simulink model "IPMSM_Motor_Drive1"  (R2022b)
settings: Solver=VariableStepAuto  StartTime=0.0  StopTime=10.0  RelTol=1e-3
InitFcn:
  | Ts=1/(16000);
  | Ts_Control=Ts;
  | Ts_Power=Ts;
  | PulseDuration=5e-6;
  | Vrefpeak=399;
  | VDC=800;
  | R=1.4;
  | L=1e-4;
  | Freq = 120;
  | Rc= 0.00001;
  | C=220e-6;
  | Ld = 473e-6;
  | Lq = 1155e-6;
  | Fpm = 0.1383;
  | Rs = 0.036;
libraries: spsIGBTDiodeLib x12, spsDiodeLib x6, spsSeriesRLCBranchLib x3, slpidlib x2, spsDCVoltageSourceLib x1, mcbcontrolslib x1, spsPermanentMagnetSynchronousMachineLib x1, simulink x1, spsThreePhaseVIMeasurementLib x1, spspowerguiLib x1
settings Model: Creator=ahmetcan.akuz  LastModifiedBy=ahmetcan.akuz

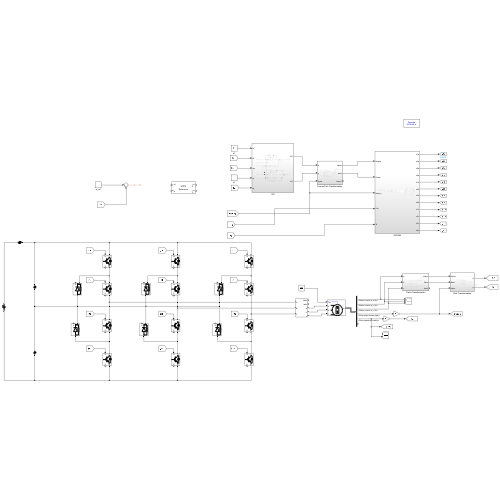
[thumbnail: Simulink's stored preview of the top-level diagram]
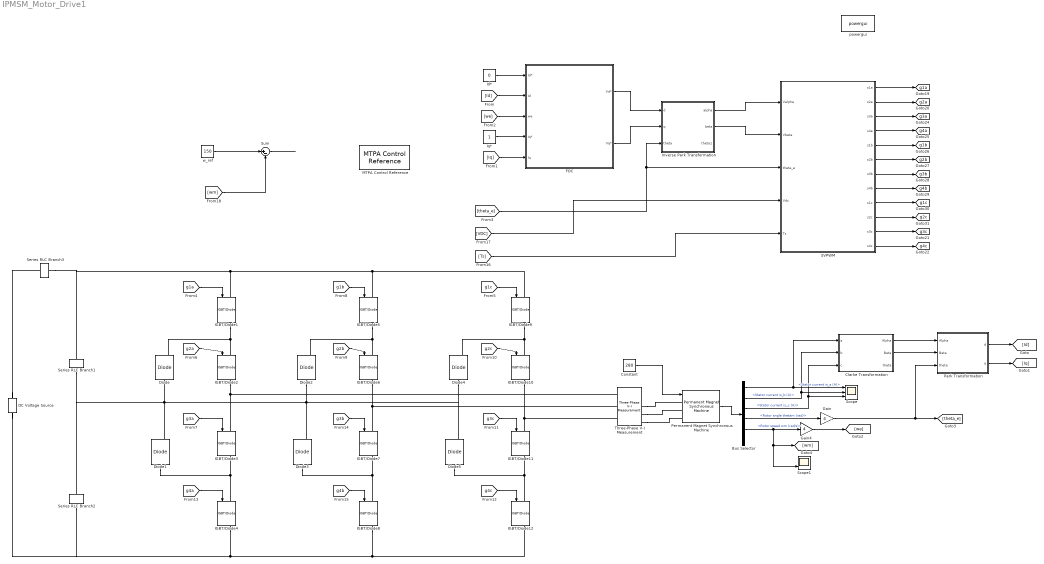
== system IPMSM_Motor_Drive1 ==
  Bus Selector : BusSelector  OutputSignals=Stator current is_a (A),Stator current is_b (A),Stator current is_c (A),Rotor angle thetam (rad),Rotor speed wm (rad/s),Electromagnetic torque Te (N*m)
  Clarke Transformation : Subsystem
  Constant : Constant  Value=280
  DC Voltage Source : spsDCVoltageSourceLib/DC Voltage Source  Amplitude=800  Measurements=None
  Diode{,1..5} (6 alike) : spsDiodeLib/Diode  Ron=1e-5  Lon=0  Vf=0.8  IC=0  UseSnubber=0  Rs=1e6  Cs=inf  Measurements=on
  FOC : Subsystem
  Gain : Gain  Gain=4
  Gain4 : Gain  Gain=4
  IGBT/Diode{1..12} (12 alike) : spsIGBTDiodeLib/IGBT//Diode  Ron=1e-3  Rs=1e5  Cs=inf  Measurements=on
  Id* : Constant  Value=0
  Inverse Park Transformation : Subsystem
  Iq* : Constant
  MTPA Control Reference : mcbcontrolslib/MTPA Control Reference  VariantSelect=Interior PMSM  polePairs=4  Rs=0.36  Ld=0.2e-3  Lq=0.4e-3  FluxPM=6.4e-3  ilimit=7.1  V_dc=24  Units=Per-Unit (PU)  N_base=4107  I_base=19.3  T_base=0.74112  N_base_disp=3182
      settings: LibrarySourceBlock=mcblib/Controls/Control Reference/MTPA Control Reference
  Park Transformation : Subsystem
  Permanent Magnet Synchronous Machine : spsPermanentMagnetSynchronousMachineLib/Permanent Magnet Synchronous Machine  NbPhases=3  FluxDistribution=Sinusoidal  RotorType=Salient-pole  MechanicalLoad=Torque Tm  PresetModel=No  ShowDetailedParameters=on  MeasurementBus=off  Resistance=0.036  Inductance=8.5e-3  dqInductances=[0.473e-3,1.155e-3]  La=0.000395  MachineConstant=Flux linkage established by magnets (V.s)  Flux=0.1383  VoltageCst=100.3394  TorqueCst=0.8298  Flat=120  Mechanical=[0.0027 0.0004924 4 0]  PolePairs=4  InitialConditions=[0,0, 0,0]  InitialConditions5ph=[0 0 0 0 0 0]  RefAngle=Aligned with phase A axis (original Park)  IterativeDiscreteModel=Trapezoidal non iterative  TsBlock=-1  TsPowergui=0
  SVPWM : Subsystem
  Scope : Scope  NumInputPorts=3
  Scope1 : Scope  NumInputPorts=2
  Series RLC Branch1 : spsSeriesRLCBranchLib/Series RLC Branch  LConnTagsString=__new0  RConnTagsString=__new0  BranchType=C  Resistance=1e-3  Inductance=1e-3  SetiL0=off  InitialCurrent=0  Capacitance=500e-6  Setx0=on  InitialVoltage=800/2  Measurements=Branch voltage
  Series RLC Branch2 : spsSeriesRLCBranchLib/Series RLC Branch  LConnTagsString=__new0  RConnTagsString=__new0  BranchType=C  Resistance=1e-3  Inductance=1e-3  SetiL0=off  InitialCurrent=0  Capacitance=500e-6  Setx0=on  InitialVoltage=800/2  Measurements=Branch voltage
  Series RLC Branch3 : spsSeriesRLCBranchLib/Series RLC Branch  LConnTagsString=__new0  RConnTagsString=__new0  BranchType=R  Resistance=1e-3  Inductance=1e-3  SetiL0=off  InitialCurrent=0  Capacitance=500e-6  Setx0=on  InitialVoltage=800/2  Measurements=Branch voltage
  Sum : Sum  Inputs=|+-
  Three-Phase V-I Measurement : spsThreePhaseVIMeasurementLib/Three-Phase V-I Measurement  VoltageMeasurement=phase-to-phase  SetLabelV=off  LabelV=Vabc  Vpu=off  VpuLL=off  CurrentMeasurement=yes  SetLabelI=off  LabelI=Iabc  Ipu=off  Pbase=100e6  Vbase=500e3  OutputType=Complex  PhasorSimulation=off  PSBequivalent=0
  powergui : spspowerguiLib/powergui  Priority=1  SimulationMode=Discrete  SampleTime=Ts/10  frequency=60  Iterations=50  frequencyindice=0  Pbase=100e6  ErrMax=1e-4  UnitsV=kV  UnitsW=MW  buscounter=0  FunctionMessages=off  echomessages=off  EnableUseOfTLC=off  CurrentSourceSwitches=off  DisableSnubberDevices=off  DisableRonSwitches=off  DisableVfSwitches=off  DisplayEquations=off  AutomaticDiscreteSolvers=off  SolverType=Tustin/Backward Euler (TBE)  Interpol=off  ExternalGateDelay=off  methode=off  Ts=100  x0status=blocks  SPID=off  SwTol=0  HookPort=off  NonlinearTolerance=1e-4  nMaxIteration=100  ContinueOnMaxIteration=off  RestoreLinks=warning  ResistiveCurrentMeasurement=off  Frange=[0:2:500]  Ylog=off  Xlog=on  ShowGrid=off  save=off  variable=ZData  structure=0  ZoomFFT=off  StartTime=0.0  cycles=1  DisplayStyle=1  fundamental=60  FreqAxis=off  MaxFrequency=1000  frequencyindicesteady=1  RmsSteady=1  display=off
  w_ref : Constant  Value=150
  tag scope: g1a=global, g1b=global, g1c=global, g2a=global, g2b=global, g2c=global, g3a=global, g3b=global, g3c=global, g4a=global, g4b=global, g4c=global
  wires:
  Permanent Magnet Synchronous Machine/1 -> Bus Selector/1
  Bus Selector/1 -> Scope/1, Clarke Transformation/1(a)  "<Stator current is_a (A)>"
  Bus Selector/2 -> Clarke Transformation/2(b), Scope/2  "<Stator current is_b (A)>"
  Bus Selector/3 -> Clarke Transformation/3(c), Scope/3  "<Stator current is_c (A)>"
  Clarke Transformation/2(Beta) -> Park Transformation/2(Beta)
  Clarke Transformation/1(Alpha) -> Park Transformation/1(Alpha)
  Bus Selector/4 -> Gain/1  "<Rotor angle thetam (rad)>"
  Gain/1 -> [theta_e], Park Transformation/3(theta)
  Park Transformation/1(d) -> [Id]
  Park Transformation/2(q) -> [Iq]
  Bus Selector/5 -> [wm], Scope1/2, Gain4/1  "<Rotor speed wm (rad/s)>"
  Gain4/1 -> [we]
  Id*/1 -> FOC/1(Id*)
  [Id] -> FOC/2(Id)
  [we] -> FOC/3(we)
  Iq*/1 -> FOC/4(Iq*)
  [Iq] -> FOC/5(Iq)
  FOC/1(Vd*) -> Inverse Park Transformation/1(d)
  FOC/2(Vq*) -> Inverse Park Transformation/2(q)
  [theta_e] -> SVPWM/3(theta_e), Inverse Park Transformation/3(theta)
  Inverse Park Transformation/1(alpha) -> SVPWM/1(Valpha)
  Inverse Park Transformation/2(beta) -> SVPWM/2(Vbeta)
  [g1a] -> IGBT/Diode1/1
  [g2b] -> IGBT/Diode6/1
  [g3b] -> IGBT/Diode7/1
  [g4b] -> IGBT/Diode8/1
  [g4a] -> IGBT/Diode4/1
  [g3a] -> IGBT/Diode3/1
  [g2a] -> IGBT/Diode2/1
  [g1b] -> IGBT/Diode5/1
  [g1c] -> IGBT/Diode9/1
  [g2c] -> IGBT/Diode10/1
  [g3c] -> IGBT/Diode11/1
  [g4c] -> IGBT/Diode12/1
  SVPWM/1(s1a) -> [g1a]
  SVPWM/2(s2a) -> [g2a]
  SVPWM/12(s4c) -> [g4c]
  SVPWM/11(s3c) -> [g3c]
  SVPWM/3(s3a) -> [g3a]
  SVPWM/4(s4a) -> [g4a]
  SVPWM/5(s1b) -> [g1b]
  SVPWM/6(s2b) -> [g2b]
  SVPWM/7(s3b) -> [g3b]
  SVPWM/8(s4b) -> [g4b]
  SVPWM/9(s1c) -> [g1c]
  SVPWM/10(s2c) -> [g2c]
  [Ts] -> SVPWM/5(Ts)
  [VDC] -> SVPWM/4(Vdc)
  Constant/1 -> Permanent Magnet Synchronous Machine/1
  w_ref/1 -> Sum/1
  [wm] -> Sum/2
  Sum/1 -> ?
  connections:
  Diode1/RConn1 -- Series RLC Branch1/RConn1 -- Series RLC Branch2/LConn1 -- Diode3/RConn1 -- Diode5/RConn1 -- Diode4/LConn1 -- Diode2/LConn1 -- Diode/LConn1
  IGBT/Diode4/LConn1 -- Diode1/LConn1 -- IGBT/Diode3/RConn1
  IGBT/Diode2/RConn1 -- IGBT/Diode3/LConn1 -- Three-Phase V-I Measurement/LConn1
  IGBT/Diode1/RConn1 -- Diode/RConn1 -- IGBT/Diode2/LConn1
  IGBT/Diode5/RConn1 -- Diode2/RConn1 -- IGBT/Diode6/LConn1
  IGBT/Diode8/LConn1 -- Diode3/LConn1 -- IGBT/Diode7/RConn1
  IGBT/Diode6/RConn1 -- Three-Phase V-I Measurement/LConn2 -- IGBT/Diode7/LConn1
  IGBT/Diode9/RConn1 -- Diode4/RConn1 -- IGBT/Diode10/LConn1
  IGBT/Diode12/LConn1 -- Diode5/LConn1 -- IGBT/Diode11/RConn1
  IGBT/Diode10/RConn1 -- Three-Phase V-I Measurement/LConn3 -- IGBT/Diode11/LConn1
  IGBT/Diode1/LConn1 -- Series RLC Branch3/LConn1 -- Series RLC Branch1/LConn1 -- IGBT/Diode9/LConn1 -- IGBT/Diode5/LConn1
  IGBT/Diode4/RConn1 -- Series RLC Branch2/RConn1 -- DC Voltage Source/LConn1 -- IGBT/Diode8/RConn1 -- IGBT/Diode12/RConn1
  Three-Phase V-I Measurement/RConn3 -- Permanent Magnet Synchronous Machine/LConn3
  Three-Phase V-I Measurement/RConn2 -- Permanent Magnet Synchronous Machine/LConn2
  Three-Phase V-I Measurement/RConn1 -- Permanent Magnet Synchronous Machine/LConn1
  DC Voltage Source/RConn1 -- Series RLC Branch3/RConn1

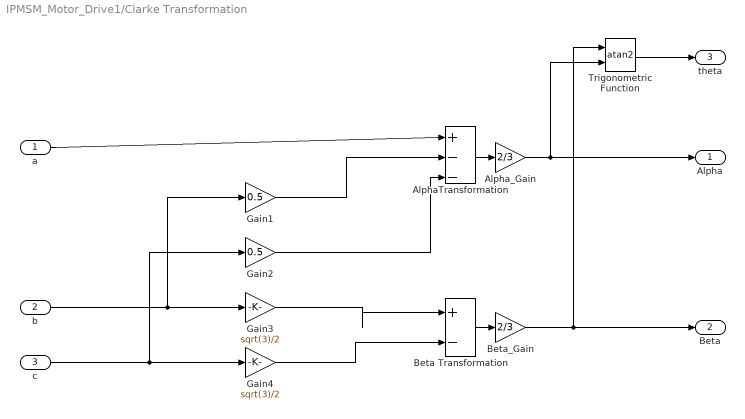
== system IPMSM_Motor_Drive1/Clarke Transformation ==
  a : Inport
  b : Inport  Port=2
  c : Inport  Port=3
  AlphaTransformation : Sum  Inputs=|+--
  Alpha_Gain : Gain  Gain=2/3
  Beta Transformation : Sum  Inputs=|+-
  Beta_Gain : Gain  Gain=2/3
  Gain1 : Gain  Gain=0.5
  Gain2 : Gain  Gain=0.5
  Gain3 : Gain  Gain=sqrt(3)/2
  Gain4 : Gain  Gain=sqrt(3)/2
  Trigonometric Function : Trigonometry  Operator=atan2
  Alpha : Outport
  Beta : Outport  Port=2
  theta : Outport  Port=3
  wires:
  Gain1/1 -> AlphaTransformation/2
  Gain4/1 -> Beta Transformation/2
  AlphaTransformation/1 -> Alpha_Gain/1
  Gain3/1 -> Beta Transformation/1
  b/1 -> Gain1/1, Gain3/1
  Gain2/1 -> AlphaTransformation/3
  c/1 -> Gain2/1, Gain4/1
  Beta Transformation/1 -> Beta_Gain/1
  a/1 -> AlphaTransformation/1
  Trigonometric Function/1 -> theta/1
  Alpha_Gain/1 -> Trigonometric Function/2, Alpha/1
  Beta_Gain/1 -> Trigonometric Function/1, Beta/1

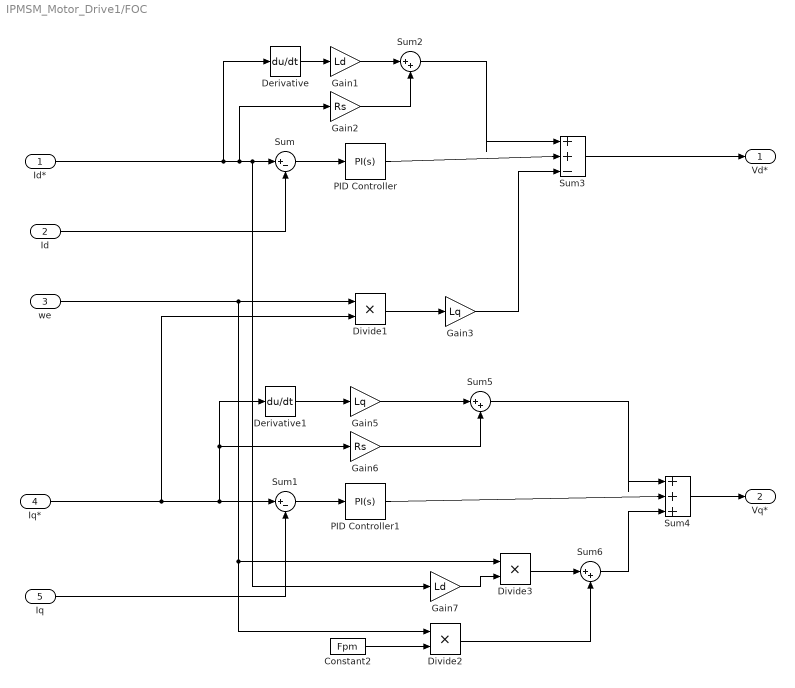
== system IPMSM_Motor_Drive1/FOC ==
  Id* : Inport
  Id : Inport  Port=2
  we : Inport  Port=3
  Iq* : Inport  Port=4
  Iq : Inport  Port=5
  Constant2 : Constant  Value=Fpm
  Derivative : Derivative
  Derivative1 : Derivative
  Divide1 : Product  Inputs=**
  Divide2 : Product  Inputs=**
  Divide3 : Product  Inputs=**
  Gain1 : Gain  Gain=Ld
  Gain2 : Gain  Gain=Rs
  Gain3 : Gain  Gain=Lq
  Gain5 : Gain  Gain=Lq
  Gain6 : Gain  Gain=Rs
  Gain7 : Gain  Gain=Ld
  PID Controller : slpidlib/PID Controller  Controller=PI  Form=Parallel  TimeDomain=Continuous-time  UseExternalTs=off  SampleTime=-1  IntegratorMethod=Forward Euler  FilterMethod=Forward Euler  ControllerParametersSource=internal  P=1  I=1  UseKiTs=off  D=0  N=100  UseFilter=on  TunerSelectOption=Transfer Function Based (PID Tuner App)  InitialConditionSource=internal  InitialConditionForIntegrator=0  InitialConditionForFilter=0  DifferentiatorICPrevScaledInput=0  ExternalReset=none  TrackingMode=off  Kt=1  LimitOutput=off  SatLimitsSource=internal  UpperSaturationLimit=inf  LowerSaturationLimit=-inf  LinearizeAsGain=on  AntiWindupMode=none  Kb=1  LimitIntegrator=off  UpperIntegratorSaturationLimit=inf  LowerIntegratorSaturationLimit=-inf  POutMin=[]  POutMax=[]  IOutMin=[]  IOutMax=[]  DOutMin=[]  DOutMax=[]  NOutMin=[]  NOutMax=[]  SumOutMin=[]  SumOutMax=[]  SaturationOutMin=[]  SaturationOutMax=[]  PParamMin=[]  PParamMax=[]  IParamMin=[]  IParamMax=[]  DParamMin=[]  DParamMax=[]  NParamMin=[]  NParamMax=[]  KbParamMin=[]  KbParamMax=[]  KtParamMin=[]  KtParamMax=[]  KbOutMin=[]  KbOutMax=[]  KtOutMin=[]  KtOutMax=[]  IntegratorOutMin=[]  IntegratorOutMax=[]  FilterOutMin=[]  FilterOutMax=[]  SumI1OutMin=[]  SumI1OutMax=[]  SumI2OutMin=[]  SumI2OutMax=[]  SumI3OutMin=[]  SumI3OutMax=[]  SumI4OutMin=[]  SumI4OutMax=[]  SumDOutMin=[]  SumDOutMax=[]  DifferentiatorOutMin=[]  DifferentiatorOutMax=[]  FilterDiffOutCoefMin=[]  FilterDiffOutCoefMax=[]  ReciprocalOutMin=[]  ReciprocalOutMax=[]  SumDenOutMin=[]  SumDenOutMax=[]  SumNumOutMin=[]  SumNumOutMax=[]  DivideOutMin=[]  DivideOutMax=[]  UdiffTsProdOutMin=[]  UdiffTsProdOutMax=[]  NTsProdOutMin=[]  NTsProdOutMax=[]  UintegralTsProdOutMin=[]  UintegralTsProdOutMax=[]  UngainTsProdOutMin=[]  UngainTsProdOutMax=[]  ClampingZeroOutDataTypeStr=Inherit: Inherit via back propagation  ClampingZeroOutMin=[]  ClampingZeroOutMax=[]  FilterDenConstantOutDataTypeStr=Inherit: Inherit via back propagation  FilterDenConstantOutMin=[]  FilterDenConstantOutMax=[]  PCopyOutDataTypeStr=Inherit: Inherit via back propagation  PCopyOutMin=[]  PCopyOutMax=[]  NCopyOutDataTypeStr=Inherit: Inherit via back propagation  NCopyOutMin=[]  NCopyOutMax=[]  IntegratorContinuousStateAttributes=''  IntegratorStateMustResolveToSignalObject=off  IntegratorRTWStateStorageClass=Auto  FilterContinuousStateAttributes=''  FilterStateMustResolveToSignalObject=off  FilterRTWStateStorageClass=Auto  ParallelPVariant=InternalParameters  IdealPVariant=Disabled  IVariant=InternalParameters  DVariant=Disabled  IntegratorVariant=Continuous  SatVariant=Disabled  AWVariant=Passthrough  PCopyVariant=Disabled  TRVariant=Disabled  FdbkBlocksVariant=Forward  IdealPFdbkVariant=Disabled  SatFdbkVariant=Disabled  DerivativeFilterVariant=Disabled  NVariant=Disabled  NCopyVariant=Disabled_SignalSpec  FilterICVariant=Disabled  IntegratorICVariant=InternalICs  ExternalResetVariant=Disabled  TRSumVariant=Passthrough  SumFdbkVariant=Disabled  SumVariant=Sum_PI  TsampFilterVariant=InternalTs  TsampNgainVariant=Passthrough  TsampIntegralVariant=Passthrough  ExternalSaturationOutDataTypeStr=Inherit: Same as second input
  PID Controller1 : slpidlib/PID Controller  Controller=PI  Form=Parallel  TimeDomain=Continuous-time  UseExternalTs=off  SampleTime=-1  IntegratorMethod=Forward Euler  FilterMethod=Forward Euler  ControllerParametersSource=internal  P=1  I=1  UseKiTs=off  D=0  N=100  UseFilter=on  TunerSelectOption=Transfer Function Based (PID Tuner App)  InitialConditionSource=internal  InitialConditionForIntegrator=0  InitialConditionForFilter=0  DifferentiatorICPrevScaledInput=0  ExternalReset=none  TrackingMode=off  Kt=1  LimitOutput=off  SatLimitsSource=internal  UpperSaturationLimit=inf  LowerSaturationLimit=-inf  LinearizeAsGain=on  AntiWindupMode=none  Kb=1  LimitIntegrator=off  UpperIntegratorSaturationLimit=inf  LowerIntegratorSaturationLimit=-inf  POutMin=[]  POutMax=[]  IOutMin=[]  IOutMax=[]  DOutMin=[]  DOutMax=[]  NOutMin=[]  NOutMax=[]  SumOutMin=[]  SumOutMax=[]  SaturationOutMin=[]  SaturationOutMax=[]  PParamMin=[]  PParamMax=[]  IParamMin=[]  IParamMax=[]  DParamMin=[]  DParamMax=[]  NParamMin=[]  NParamMax=[]  KbParamMin=[]  KbParamMax=[]  KtParamMin=[]  KtParamMax=[]  KbOutMin=[]  KbOutMax=[]  KtOutMin=[]  KtOutMax=[]  IntegratorOutMin=[]  IntegratorOutMax=[]  FilterOutMin=[]  FilterOutMax=[]  SumI1OutMin=[]  SumI1OutMax=[]  SumI2OutMin=[]  SumI2OutMax=[]  SumI3OutMin=[]  SumI3OutMax=[]  SumI4OutMin=[]  SumI4OutMax=[]  SumDOutMin=[]  SumDOutMax=[]  DifferentiatorOutMin=[]  DifferentiatorOutMax=[]  FilterDiffOutCoefMin=[]  FilterDiffOutCoefMax=[]  ReciprocalOutMin=[]  ReciprocalOutMax=[]  SumDenOutMin=[]  SumDenOutMax=[]  SumNumOutMin=[]  SumNumOutMax=[]  DivideOutMin=[]  DivideOutMax=[]  UdiffTsProdOutMin=[]  UdiffTsProdOutMax=[]  NTsProdOutMin=[]  NTsProdOutMax=[]  UintegralTsProdOutMin=[]  UintegralTsProdOutMax=[]  UngainTsProdOutMin=[]  UngainTsProdOutMax=[]  ClampingZeroOutDataTypeStr=Inherit: Inherit via back propagation  ClampingZeroOutMin=[]  ClampingZeroOutMax=[]  FilterDenConstantOutDataTypeStr=Inherit: Inherit via back propagation  FilterDenConstantOutMin=[]  FilterDenConstantOutMax=[]  PCopyOutDataTypeStr=Inherit: Inherit via back propagation  PCopyOutMin=[]  PCopyOutMax=[]  NCopyOutDataTypeStr=Inherit: Inherit via back propagation  NCopyOutMin=[]  NCopyOutMax=[]  IntegratorContinuousStateAttributes=''  IntegratorStateMustResolveToSignalObject=off  IntegratorRTWStateStorageClass=Auto  FilterContinuousStateAttributes=''  FilterStateMustResolveToSignalObject=off  FilterRTWStateStorageClass=Auto  ParallelPVariant=InternalParameters  IdealPVariant=Disabled  IVariant=InternalParameters  DVariant=Disabled  IntegratorVariant=Continuous  SatVariant=Disabled  AWVariant=Passthrough  PCopyVariant=Disabled  TRVariant=Disabled  FdbkBlocksVariant=Forward  IdealPFdbkVariant=Disabled  SatFdbkVariant=Disabled  DerivativeFilterVariant=Disabled  NVariant=Disabled  NCopyVariant=Disabled_SignalSpec  FilterICVariant=Disabled  IntegratorICVariant=InternalICs  ExternalResetVariant=Disabled  TRSumVariant=Passthrough  SumFdbkVariant=Disabled  SumVariant=Sum_PI  TsampFilterVariant=InternalTs  TsampNgainVariant=Passthrough  TsampIntegralVariant=Passthrough  ExternalSaturationOutDataTypeStr=Inherit: Same as second input
  Sum : Sum  Inputs=|+-
  Sum1 : Sum  Inputs=|+-
  Sum2 : Sum  Inputs=|++
  Sum3 : Sum  Inputs=|++-
  Sum4 : Sum  Inputs=|+++
  Sum5 : Sum  Inputs=|++
  Sum6 : Sum  Inputs=|++
  Vd* : Outport
  Vq* : Outport  Port=2
  wires:
  Sum/1 -> PID Controller/1
  Iq*/1 -> Divide1/2, Gain6/1, Derivative1/1, Sum1/1
  Divide3/1 -> Sum6/1
  Id*/1 -> Derivative/1, Gain2/1, Gain7/1, Sum/1
  Derivative1/1 -> Gain5/1
  Sum6/1 -> Sum4/3
  Sum3/1 -> Vd*/1
  Gain7/1 -> Divide3/2
  Derivative/1 -> Gain1/1
  Gain1/1 -> Sum2/1
  PID Controller1/1 -> Sum4/2
  Gain2/1 -> Sum2/2
  Id/1 -> Sum/2
  Sum1/1 -> PID Controller1/1
  Sum5/1 -> Sum4/1
  Sum4/1 -> Vq*/1
  Gain6/1 -> Sum5/2
  PID Controller/1 -> Sum3/2
  Sum2/1 -> Sum3/1
  we/1 -> Divide3/1, Divide2/1, Divide1/1
  Iq/1 -> Sum1/2
  Divide2/1 -> Sum6/2
  Gain5/1 -> Sum5/1
  Constant2/1 -> Divide2/2
  Divide1/1 -> Gain3/1
  Gain3/1 -> Sum3/3

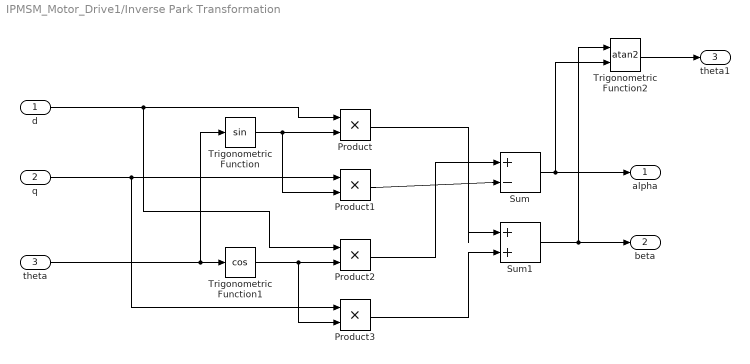
== system IPMSM_Motor_Drive1/Inverse Park Transformation ==
  d : Inport
  q : Inport  Port=2
  theta : Inport  Port=3
  Product{,1..3} (4 alike) : Product
  Sum : Sum  Inputs=|+-
  Sum1 : Sum  Inputs=|++
  Trigonometric Function : Trigonometry
  Trigonometric Function1 : Trigonometry  Operator=cos
  Trigonometric Function2 : Trigonometry  Operator=atan2
  alpha : Outport
  beta : Outport  Port=2
  theta1 : Outport  Port=3
  wires:
  Product/1 -> Sum1/1
  Trigonometric Function/1 -> Product1/2, Product/2
  d/1 -> Product2/1, Product/1
  Product2/1 -> Sum/1
  theta/1 -> Trigonometric Function/1, Trigonometric Function1/1
  Product1/1 -> Sum/2
  Trigonometric Function1/1 -> Product2/2, Product3/2
  q/1 -> Product3/1, Product1/1
  Product3/1 -> Sum1/2
  Sum/1 -> Trigonometric Function2/2, alpha/1
  Trigonometric Function2/1 -> theta1/1
  Sum1/1 -> Trigonometric Function2/1, beta/1

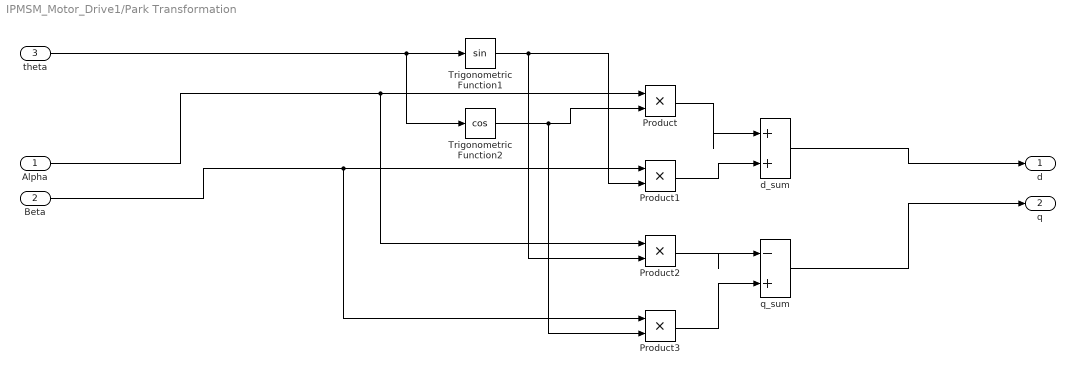
== system IPMSM_Motor_Drive1/Park Transformation ==
  Alpha : Inport
  Beta : Inport  Port=2
  theta : Inport  Port=3
  Product{,1..3} (4 alike) : Product
  Trigonometric Function1 : Trigonometry
  Trigonometric Function2 : Trigonometry  Operator=cos
  d_sum : Sum  Inputs=|++
  q_sum : Sum  Inputs=|-+
  d : Outport
  q : Outport  Port=2
  wires:
  Trigonometric Function1/1 -> Product2/2, Product1/2
  Product/1 -> d_sum/1
  Product2/1 -> q_sum/1
  Beta/1 -> Product3/1, Product1/1
  Alpha/1 -> Product2/1, Product/1
  Product3/1 -> q_sum/2
  Trigonometric Function2/1 -> Product3/2, Product/2
  Product1/1 -> d_sum/2
  q_sum/1 -> q/1
  d_sum/1 -> d/1
  theta/1 -> Trigonometric Function2/1, Trigonometric Function1/1

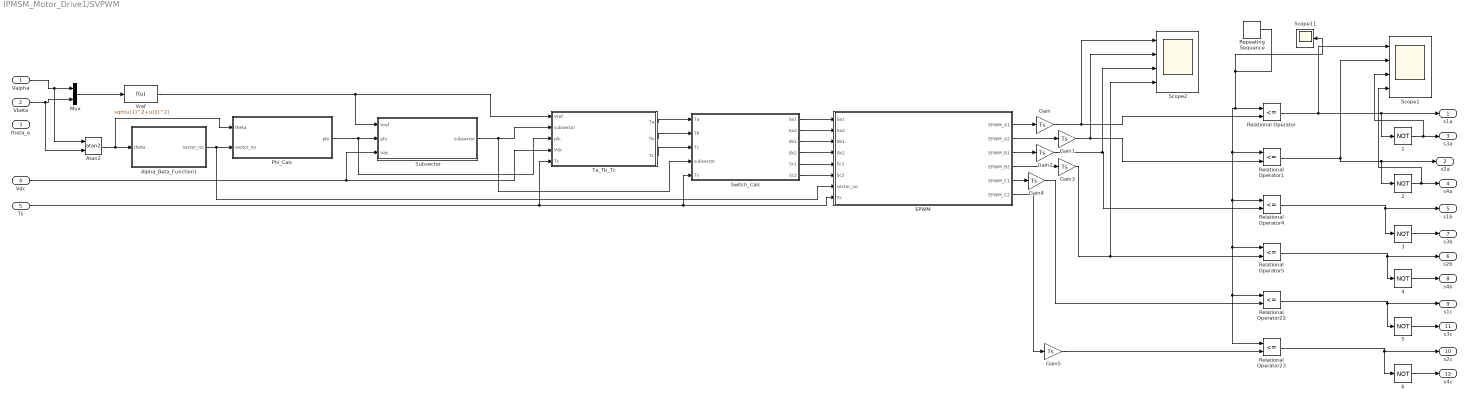
== system IPMSM_Motor_Drive1/SVPWM ==
  Valpha : Inport
  Vbeta : Inport  Port=2
  theta_e : Inport  Port=3
  Vdc : Inport  Port=4
  Ts : Inport  Port=5
  {1..6} (6 alike) : Logic  Operator=NOT  AllPortsSameDT=off  OutDataTypeStr=boolean
  Alpha_Beta_Function1 : MATLAB Function  TreatAsAtomicUnit=on
  Atan2 : Trigonometry  Operator=atan2
  EPWM : MATLAB Function  TreatAsAtomicUnit=on
  Gain{,1..5} (6 alike) : Gain  Gain=Ts
  Mux : Mux  Inputs=2
  Phi_Calc : MATLAB Function  TreatAsAtomicUnit=on
  Relational Operator{,1,4..5,22..23} (6 alike) : RelationalOperator  Operator=<=  OutDataTypeStr=boolean  InputSameDT=off
  Repeating Sequence : simulink/Sources/Repeating Sequence  rep_seq_t=[0 1 2]*[1/6000]  rep_seq_y=[0 0.01 0]
  Scope1 : Scope  NumInputPorts=4
  Scope11 : Scope
  Scope2 : Scope  NumInputPorts=4
  Subsector : MATLAB Function  TreatAsAtomicUnit=on
  Switch_Calc : MATLAB Function  TreatAsAtomicUnit=on
  Ta_Tb_Tc : MATLAB Function  TreatAsAtomicUnit=on
  Vref : Fcn  Expr=sqrt(u(1)^2+u(2)^2)
  s1a : Outport
  s2a : Outport  Port=2
  s3a : Outport  Port=3
  s4a : Outport  Port=4
  s1b : Outport  Port=5
  s2b : Outport  Port=6
  s3b : Outport  Port=7
  s4b : Outport  Port=8
  s1c : Outport  Port=9
  s2c : Outport  Port=10
  s3c : Outport  Port=11
  s4c : Outport  Port=12
  wires:
  Mux/1 -> Vref/1
  Vref/1 -> Subsector/1(Vref), Ta_Tb_Tc/1(Vref)
  Vbeta/1 -> Atan2/2, Mux/2
  Valpha/1 -> Atan2/1, Mux/1
  Atan2/1 -> Phi_Calc/1(theta), Alpha_Beta_Function1/1(theta)
  Alpha_Beta_Function1/1(sector_no) -> EPWM/7(sector_no), Phi_Calc/2(sector_no)
  Ta_Tb_Tc/2(Tb) -> Switch_Calc/2(Tb)
  Ta_Tb_Tc/3(Tc) -> Switch_Calc/3(Tc)
  Ta_Tb_Tc/1(Ta) -> Switch_Calc/1(Ta)
  Phi_Calc/1(phi) -> Ta_Tb_Tc/3(phi), Subsector/2(phi)
  Subsector/1(subsector) -> Switch_Calc/4(subsector), Ta_Tb_Tc/2(subsector)
  Vdc/1 -> Subsector/3(Vdc), Ta_Tb_Tc/4(Vdc)
  Ts/1 -> Ta_Tb_Tc/5(Ts), EPWM/8(Ts), Switch_Calc/5(Ts)
  Switch_Calc/1(Sa1) -> EPWM/1(Sa1)
  Switch_Calc/2(Sa2) -> EPWM/2(Sa2)
  Switch_Calc/3(Sb1) -> EPWM/3(Sb1)
  Switch_Calc/4(Sb2) -> EPWM/4(Sb2)
  Switch_Calc/5(Sc1) -> EPWM/5(Sc1)
  Switch_Calc/6(Sc2) -> EPWM/6(Sc2)
  Relational Operator/1 -> Scope1/1, s1a/1, 1/1
  EPWM/5(EPWM_C1) -> Gain4/1
  5/1 -> s3c/1
  6/1 -> s4c/1
  1/1 -> Scope1/3, s3a/1
  EPWM/1(EPWM_A1) -> Gain/1
  EPWM/2(EPWM_A2) -> Gain1/1
  Relational Operator23/1 -> s2c/1, 6/1
  Relational Operator22/1 -> s1c/1, 5/1
  2/1 -> Scope1/4, s4a/1
  Relational Operator1/1 -> s2a/1, 2/1, Scope1/2
  Repeating Sequence/1 -> Relational Operator/1, Relational Operator23/1, Relational Operator22/1, Relational Operator5/1, Relational Operator4/1, Relational Operator1/1, Scope11/1
  EPWM/4(EPWM_B2) -> Gain3/1
  Relational Operator5/1 -> s2b/1, 4/1
  Relational Operator4/1 -> s1b/1, 3/1
  4/1 -> s4b/1
  3/1 -> s3b/1
  EPWM/3(EPWM_B1) -> Gain2/1
  EPWM/6(EPWM_C2) -> Gain5/1
  Gain/1 -> Scope2/1, Relational Operator/2
  Gain1/1 -> Scope2/2, Relational Operator1/2
  Gain2/1 -> Scope2/3, Relational Operator4/2
  Gain3/1 -> Scope2/4, Relational Operator5/2
  Gain4/1 -> Relational Operator22/2
  Gain5/1 -> Relational Operator23/2

== matlab function IPMSM_Motor_Drive1/SVPWM/Alpha_Beta_Function1 ==
  data: theta input; sector_no output
function sector_no = fcn(theta)
sector_no=0;
if (theta>=0) && (theta<pi/3)
    sector_no=1;
end
if (theta>=pi/3) && (theta<2*pi/3)
    sector_no=2;
end
if (theta>=2*pi/3) && (theta<pi)
    sector_no=3;
end
if (theta>=-pi/3) && (theta<0)
    sector_no=6;
end
if (theta>=-2*pi/3) && (theta<-pi/3)
    sector_no=5;
end
if (theta>=-pi) && (theta<-2*pi/3)
    sector_no=4;
end
end

== matlab function IPMSM_Motor_Drive1/SVPWM/Phi_Calc ==
  data: theta input; phi output; sector_no input
function phi = fcn(theta, sector_no)
phi=0;
if (sector_no==1)
    phi=theta;
end

if (sector_no==2)
    phi=theta-pi/3;
end

if (sector_no==3)
    phi=theta-2*pi/3;
end

if (sector_no==6)
    phi=theta+pi/3;
end

if (sector_no==5)
    phi=theta+2*pi/3;
end

if (sector_no==4)
    phi=theta+pi;
end
end

== matlab function IPMSM_Motor_Drive1/SVPWM/Subsector ==
  data: Vref input; subsector output; phi input; Vdc input
function subsector = fcn(Vref, phi, Vdc)
subsector=0;
n=Vref/(2/3*Vdc);
m1=n*2/sqrt(3)*(sin(pi/3-phi));
m2=n*2/sqrt(3)*sin(phi);
if (m1<0.5) && (m2<0.5) && (m1+m2<0.5)
    subsector=1;
end
if (m1<0.5) && (m2<0.5) && (m1+m2>0.5)
    subsector=2;
end
if (m1>0.5)
    subsector=4;
end
if (m2>0.5)
    subsector=3;
end

end

== matlab function IPMSM_Motor_Drive1/SVPWM/Ta_Tb_Tc ==
  data: Vref input; subsector input; Ta output; phi input; Vdc input; Ts input; Tb output; Tc output
function [Ta, Tb, Tc] = fcn(Vref, subsector, phi, Vdc, Ts)
Ta=0; 
Tb=0; 
Tc=0;

m=Vref/(2/3*Vdc);
k=2/sqrt(3)*m*Ts;

if (subsector==1)
        Ta=2*k*sin(pi/3-phi);
        Tb=Ts-2*k*sin(pi/3+phi);
        Tc=2*k*sin(phi);
end
if (subsector==2)
        Ta=Ts-2*k*sin(phi);
        Tb=2*k*sin(pi/3+phi)-Ts;
        Tc=Ts-2*k*sin(pi/3-phi);
end
if (subsector==3)
        Ta=2*k*sin(phi)-Ts;
        Tb=2*k*sin(pi/3-phi);
        Tc=2*Ts-2*k*sin(pi/3+phi);
end
if (subsector==4)
        Ta=2*Ts-2*k*sin(pi/3+phi);
        Tb=2*k*sin(phi);
        Tc=2*k*sin(pi/3-phi)-Ts;
end

end

== matlab function IPMSM_Motor_Drive1/SVPWM/Switch_Calc ==
  data: Ta input; Tb input; Sa1 output; Tc input; Sa2 output; Sb1 output; Sb2 output; Sc1 output; Sc2 output; subsector input; Ts input
function [Sa1, Sa2, Sb1, Sb2, Sc1, Sc2] = fcn(Ta, Tb, Tc, subsector, Ts)
Sa1=0; Sa2=0;
Sb1=0; Sb2=0;
Sc1=0; Sc2=0;

if (subsector==1)
       Sa1=(Tc+Ta)/4;
       Sa2=Ts/2;
       Sb1=Tc/4;
       Sb2=Ts/2-Ta/4;
       Sc1=0;
       Sc2=Ts/2-Ta/4-Tc/4;
end
if (subsector==2)
       Sa1=(Ta+Tc)/4+Tb/2;
       Sa2=Ts/2;
       Sb1=Tc/4;
       Sb2=Ts/2-Ta/4;
       Sc1=0;
       Sc2=(Ta+Tc)/4;
end
if (subsector==3)
       Sa1=Ts/2-Tc/4;
       Sa2=Ts/2;
       Sb1=Ta/2+Tc/4;
       Sb2=Ts/2;
       Sc1=0;
       Sc2=Tc/4;
end
if (subsector==4)
       Sa1=Ts/2-Ta/4;
       Sa2=Ts/2;
       Sb1=0;
       Sb2=Ta/4+Tb/2;
       Sc1=0;
       Sc2=Ta/4;
end
end

== matlab function IPMSM_Motor_Drive1/SVPWM/EPWM ==
  data: Sa1 input; Sa2 input; EPWM_A1 output; Sb1 input; EPWM_A2 output; EPWM_B1 output; EPWM_B2 output; EPWM_C1 output; EPWM_C2 output; Sb2 input; Sc1 input; Sc2 input; sector_no input; Ts input
% Bu koddaki kaydırma ve Ts/2ler pek kafama yatmadı.

function [EPWM_A1, EPWM_A2, EPWM_B1, EPWM_B2, EPWM_C1, EPWM_C2] = fcn(Sa1, Sa2, Sb1, Sb2, Sc1, Sc2, sector_no, Ts)
EPWM_A1=0; EPWM_A2=0;
EPWM_B1=0; EPWM_B2=0;
EPWM_C1=0; EPWM_C2=0;


if (sector_no==1)
        EPWM_A1=Sa1; EPWM_A2=Sa2;
        EPWM_B1=Sb1; EPWM_B2=Sb2;
        EPWM_C1=Sc1; EPWM_C2=Sc2;
end
if (sector_no==2)
        EPWM_A1=Ts/2-Sb2; EPWM_A2=Ts/2-Sb1;
        EPWM_B1=Ts/2-Sc2; EPWM_B2=Ts/2-Sc1;
        EPWM_C1=Ts/2-Sa2; EPWM_C2=Ts/2-Sa1;
end
if (sector_no==3)
        EPWM_A1=Sc1; EPWM_A2=Sc2;
        EPWM_B1=Sa1; EPWM_B2=Sa2;
        EPWM_C1=Sb1; EPWM_C2=Sb2;
end
if (sector_no==4)
        EPWM_A1=Ts/2-Sa2; EPWM_A2=Ts/2-Sa1;
        EPWM_B1=Ts/2-Sb2; EPWM_B2=Ts/2-Sb1;
        EPWM_C1=Ts/2-Sc2; EPWM_C2=Ts/2-Sc1;    
end
if (sector_no==5)
        EPWM_A1=Sb1; EPWM_A2=Sb2;
        EPWM_B1=Sc1; EPWM_B2=Sc2;
        EPWM_C1=Sa1; EPWM_C2=Sa2;
end
if (sector_no==6)
        EPWM_A1=Ts/2-Sc2; EPWM_A2=Ts/2-Sc1;
        EPWM_B1=Ts/2-Sa2; EPWM_B2=Ts/2-Sa1;
        EPWM_C1=Ts/2-Sb2; EPWM_C2=Ts/2-Sb1;
end
end
